simulink model "mechanics_with_estimation"  (R2014a)
settings: Solver=ode2  StartTime=0.0  StopTime=10  FixedStep=0.001  RelTol=1e-3
InitFcn:
  | estimation_initfcn
values from neighbouring files (symbols this model uses):
  c = [x y z]'    [estimation_initfcn.m]
  I_xx = 1/12*m*(y^2+z^2)    (= 0.00181666666667)    [estimation_initfcn.m]
  I_yy = 1/12*m*(x^2+z^2)    (= 0.0418166666667)    [estimation_initfcn.m]
  I_zz = 1/12*m*(y^2+x^2)    (= 0.0433333333333)    [estimation_initfcn.m]
  m = 2    [estimation_initfcn.m]
  x = 0.5    [estimation_initfcn.m]
  y = 0.1    [estimation_initfcn.m]
  z = 0.03    [estimation_initfcn.m]
undefined symbols (not defined in the file or in its folder): X, Y, Z
libraries: nesl_utility x16, sm_lib x11
settings Model: Creator=wirnshofer  LastModifiedBy=benediktibk

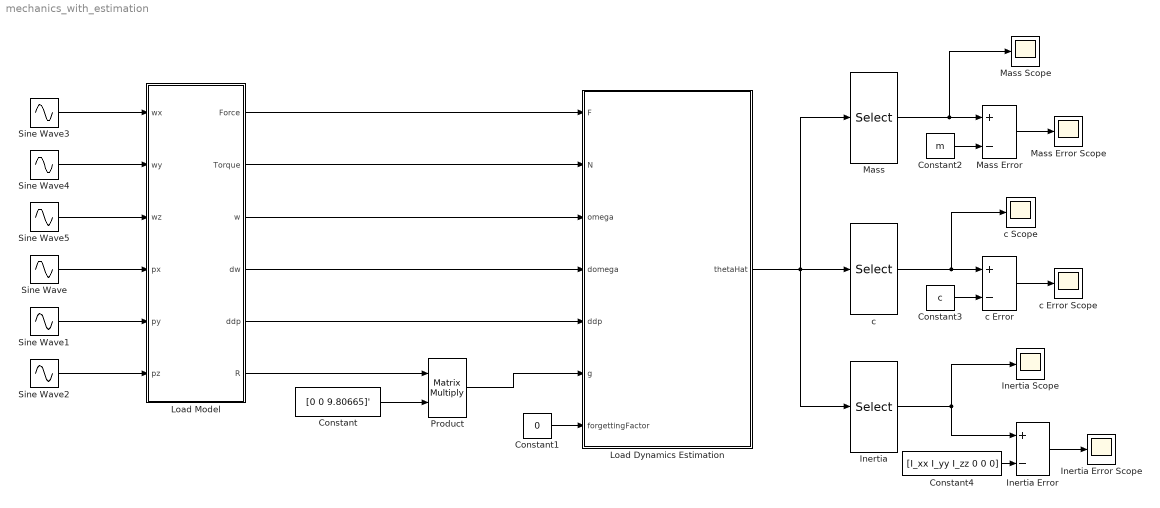
== system mechanics_with_estimation ==
  Constant : Constant  Value=[0 0 9.80665]'
  Constant1 : Constant  Value=0
  Constant2 : Constant  Value=m
  Constant3 : Constant  Value=c
  Constant4 : Constant  Value=[I_xx I_yy I_zz 0 0 0]
  Inertia : Selector  InputPortWidth=10  Indices=[5:10]
  Inertia Error : Sum  Inputs=+-
  Inertia Error Scope : Scope
      settings: ShowLegends=on  TimeRange=10  YMin=-0.9141621971570832  YMax=1.017206776816391  SaveName=ScopeData5
  Inertia Scope : Scope
      settings: ShowLegends=on  TimeRange=10  YMin=-1.003242729679008  YMax=1.975338173027628  SaveName=ScopeData2
  Load Dynamics Estimation : MATLAB Function  TreatAsAtomicUnit=on
  Load Model : Subsystem
  Mass : Selector  InputPortWidth=10
  Mass Error : Sum  Inputs=+-
  Mass Error Scope : Scope
      settings: ShowLegends=on  TimeRange=10  YMin=-0.2  YMax=0.15  SaveName=ScopeData3
  Mass Scope : Scope
      settings: ShowLegends=on  TimeRange=10  YMin=1.85  YMax=2.2
  Product : Product  Multiplication=Matrix(*)
  Sine Wave : Sin  Amplitude=0.2  Frequency=5  SampleTime=0
  Sine Wave1 : Sin  Amplitude=0.3  Frequency=4  SampleTime=0
  Sine Wave2 : Sin  Amplitude=0.2  Frequency=10  SampleTime=0
  Sine Wave3 : Sin  Amplitude=pi/4*1  Frequency=3  SampleTime=0
  Sine Wave4 : Sin  Amplitude=0.6  Frequency=8  SampleTime=0
  Sine Wave5 : Sin  Frequency=7  SampleTime=0
  c : Selector  InputPortWidth=10  Indices=[2:4]
  c Error : Sum  Inputs=+-
  c Error Scope : Scope
      settings: ShowLegends=on  TimeRange=10  YMin=-1.893593468040734  YMax=2.453897654456469  SaveName=ScopeData4
  c Scope : Scope
      settings: ShowLegends=on  TimeRange=10  YMin=-4.148671096345517  YMax=2.039036544850497
  wires:
  Constant/1 -> Product/2
  Product/1 -> Load Dynamics Estimation/6(g)
  Constant1/1 -> Load Dynamics Estimation/7(forgettingFactor)
  Sine Wave3/1 -> Load Model/1(wx)
  Sine Wave4/1 -> Load Model/2(wy)
  Sine Wave5/1 -> Load Model/3(wz)
  Sine Wave/1 -> Load Model/4(px)
  Sine Wave1/1 -> Load Model/5(py)
  Sine Wave2/1 -> Load Model/6(pz)
  Load Model/1(Force) -> Load Dynamics Estimation/1(F)
  Load Model/2(Torque) -> Load Dynamics Estimation/2(N)
  Load Model/3(w) -> Load Dynamics Estimation/3(omega)
  Load Model/4(dw) -> Load Dynamics Estimation/4(domega)
  Load Model/5(ddp) -> Load Dynamics Estimation/5(ddp)
  Load Model/6(R) -> Product/1
  Mass/1 -> Mass Error/1, Mass Scope/1
  Load Dynamics Estimation/1(thetaHat) -> Inertia/1, Mass/1, c/1
  c/1 -> c Error/1, c Scope/1
  Inertia/1 -> Inertia Error/1, Inertia Scope/1
  Constant2/1 -> Mass Error/2
  Mass Error/1 -> Mass Error Scope/1
  Constant3/1 -> c Error/2
  c Error/1 -> c Error Scope/1
  Constant4/1 -> Inertia Error/2
  Inertia Error/1 -> Inertia Error Scope/1

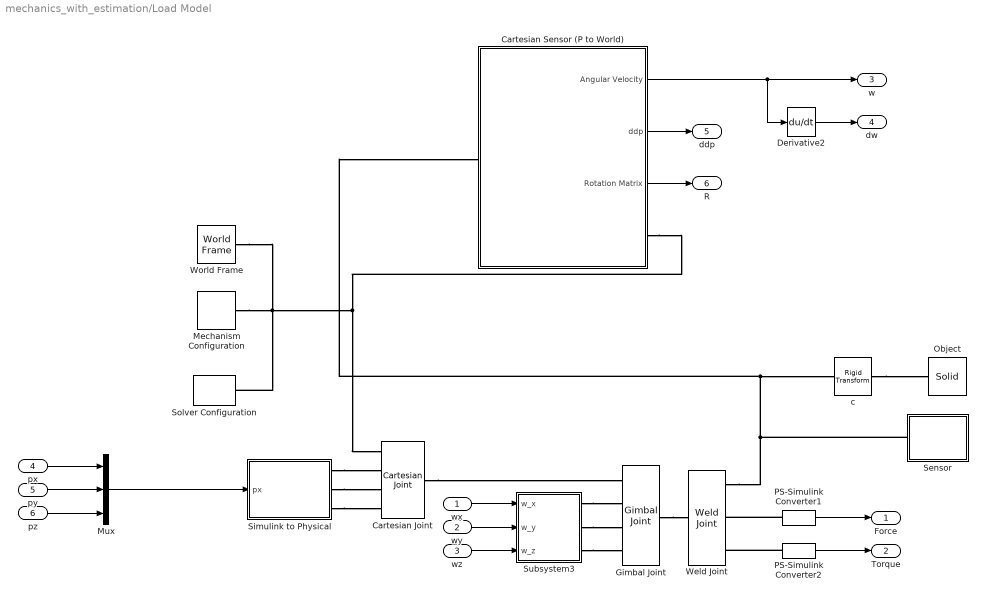
== system mechanics_with_estimation/Load Model ==
  wx : Inport
  wy : Inport  Port=2
  wz : Inport  Port=3
  px : Inport  Port=4
  py : Inport  Port=5
  pz : Inport  Port=6
  Cartesian Joint : sm_lib/Joints/Cartesian Joint  SenseConstraintForce=off  SenseConstraintForceX=off  SenseConstraintForceY=off  SenseConstraintForceZ=off  SenseConstraintTorque=off  SenseConstraintTorqueX=off  SenseConstraintTorqueY=off  SenseConstraintTorqueZ=off  SenseTotalForce=off  SenseTotalForceX=off  SenseTotalForceY=off  SenseTotalForceZ=off  SenseTotalTorque=off  SenseTotalTorqueX=off  SenseTotalTorqueY=off  SenseTotalTorqueZ=off  CompositeWrenchDir=FollowerOnBase  CompositeWrenchFrame=BaseFrame  PxEquilibriumPosition=0  PxEquilibriumPositionUnits=m  PxSpringStiffness=0  PxSpringStiffnessUnits=N/m  PxDampingCoefficient=0  PxDampingCoefficientUnits=N/(m/s)  PxTorqueActuationMode=ComputedTorque  PxMotionActuationMode=InputMotion  PxSensePosition=off  PxSenseVelocity=off  PxSenseAcceleration=off  PxSenseTorqueForce=off  PxPositionTargetValue=0  PxPositionTargetValueUnits=m  PxPositionTargetSpecify=off  PxPositionTargetPriority=High  PxVelocityTargetValue=0  PxVelocityTargetValueUnits=m/s  PxVelocityTargetSpecify=off  PxVelocityTargetPriority=High  PyEquilibriumPosition=0  PyEquilibriumPositionUnits=m  PySpringStiffness=0  PySpringStiffnessUnits=N/m  PyDampingCoefficient=0  PyDampingCoefficientUnits=N/(m/s)  PyTorqueActuationMode=ComputedTorque  PyMotionActuationMode=InputMotion  PySensePosition=off  PySenseVelocity=off  PySenseAcceleration=off  PySenseTorqueForce=off  PyPositionTargetValue=0  PyPositionTargetValueUnits=m  PyPositionTargetSpecify=off  PyPositionTargetPriority=High  PyVelocityTargetValue=0  PyVelocityTargetValueUnits=m/s  PyVelocityTargetSpecify=off  PyVelocityTargetPriority=High  PzEquilibriumPosition=0  PzEquilibriumPositionUnits=m  PzSpringStiffness=0  PzSpringStiffnessUnits=N/m  PzDampingCoefficient=0  PzDampingCoefficientUnits=N/(m/s)  PzTorqueActuationMode=ComputedTorque  PzMotionActuationMode=InputMotion  PzSensePosition=off  PzSenseVelocity=off  PzSenseAcceleration=off  PzSenseTorqueForce=off  PzPositionTargetValue=0  PzPositionTargetValueUnits=m  PzPositionTargetSpecify=off  PzPositionTargetPriority=High  PzVelocityTargetValue=0  PzVelocityTargetValueUnits=m/s  PzVelocityTargetSpecify=off  PzVelocityTargetPriority=High  BlockFunction=simmechanics.library.joints.cartesian_joint
  Cartesian Sensor (P to World) : Subsystem
  Derivative2 : Derivative
  Gimbal Joint : sm_lib/Joints/Gimbal Joint  SenseConstraintForce=off  SenseConstraintForceX=off  SenseConstraintForceY=off  SenseConstraintForceZ=off  SenseConstraintTorque=off  SenseConstraintTorqueX=off  SenseConstraintTorqueY=off  SenseConstraintTorqueZ=off  SenseTotalForce=off  SenseTotalForceX=off  SenseTotalForceY=off  SenseTotalForceZ=off  SenseTotalTorque=off  SenseTotalTorqueX=off  SenseTotalTorqueY=off  SenseTotalTorqueZ=off  CompositeWrenchDir=FollowerOnBase  CompositeWrenchFrame=BaseFrame  RxEquilibriumPosition=0  RxEquilibriumPositionUnits=deg  RxSpringStiffness=0  RxSpringStiffnessUnits=N*m/deg  RxDampingCoefficient=0  RxDampingCoefficientUnits=N*m/(deg/s)  RxTorqueActuationMode=ComputedTorque  RxMotionActuationMode=InputMotion  RxSensePosition=off  RxSenseVelocity=off  RxSenseAcceleration=off  RxSenseTorqueForce=off  RxPositionTargetValue=0  RxPositionTargetValueUnits=deg  RxPositionTargetSpecify=off  RxPositionTargetPriority=High  RxVelocityTargetValue=0  RxVelocityTargetValueUnits=deg/s  RxVelocityTargetSpecify=off  RxVelocityTargetPriority=High  RyEquilibriumPosition=0  RyEquilibriumPositionUnits=deg  RySpringStiffness=0  RySpringStiffnessUnits=N*m/deg  RyDampingCoefficient=0  RyDampingCoefficientUnits=N*m/(deg/s)  RyTorqueActuationMode=ComputedTorque  RyMotionActuationMode=InputMotion  RySensePosition=off  RySenseVelocity=off  RySenseAcceleration=off  RySenseTorqueForce=off  RyPositionTargetValue=0  RyPositionTargetValueUnits=deg  RyPositionTargetSpecify=off  RyPositionTargetPriority=High  RyVelocityTargetValue=0  RyVelocityTargetValueUnits=deg/s  RyVelocityTargetSpecify=off  RyVelocityTargetPriority=High  RzEquilibriumPosition=0  RzEquilibriumPositionUnits=deg  RzSpringStiffness=0  RzSpringStiffnessUnits=N*m/deg  RzDampingCoefficient=0  RzDampingCoefficientUnits=N*m/(deg/s)  RzTorqueActuationMode=ComputedTorque  RzMotionActuationMode=InputMotion  RzSensePosition=off  RzSenseVelocity=off  RzSenseAcceleration=off  RzSenseTorqueForce=off  RzPositionTargetValue=0  RzPositionTargetValueUnits=deg  RzPositionTargetSpecify=off  RzPositionTargetPriority=High  RzVelocityTargetValue=0  RzVelocityTargetValueUnits=deg/s  RzVelocityTargetSpecify=off  RzVelocityTargetPriority=High  BlockFunction=simmechanics.library.joints.gimbal_joint
  Mechanism Configuration : sm_lib/Utilities/Mechanism Configuration  UniformGravity=Constant  GravityVector=[0 0 -9.80665]  GravityUnits=m/s^2  LinearizationDelta=0.001  BlockFunction=simmechanics.library.utilities.mechanism_configuration
  Mux : Mux  Inputs=3
  Object : sm_lib/Body Elements/Solid  InertiaType=Custom  Mass=m  MassUnits=kg  CenterOfMass=[0 0 0]  CenterOfMassUnits=m  MomentsOfInertia=[I_xx I_yy I_zz]  MomentsOfInertiaUnits=kg*m^2  ProductsOfInertia=[0 0 0]  ProductsOfInertiaUnits=kg*m^2  DensityBased=on  Density=1000  DensityUnits=kg/(m^3)  GraphicType=FromGeometry  MarkerShape=Sphere  MarkerSize=10  MarkerSizeUnits=m  GraphicVisPropType=SimpleVisualProperties  GraphicDiffuseColor=[0.5 0.5 0.5]  GraphicSpecularColor=[0.5 0.5 0.5 1.0]  GraphicAmbientColor=[0.15 0.15 0.15 1.0]  GraphicEmissiveColor=[0.0 0.0 0.0 1.0]  GraphicShininess=75  GraphicOpacity=1.0  GeometryShape=Brick  RectangleSize=[1 1]  RectangleSizeUnits=m  BrickDimensions=[x y z]  BrickDimensionUnits=m  CylinderRadius=1  CylinderRadiusUnits=m  CylinderLength=1  CylinderLengthUnits=m  SphereRadius=1  SphereRadiusUnits=m  EllipsoidRadii=[1 1 1]  EllipsoidRadiiUnits=m  ExtrusionCrossSection=[1 1; -1 1; -1 -1; 1 -1]  ExtrusionCrossSectionUnits=m  ExtrusionLength=1  ExtrusionLengthUnits=m  PolygonNumSides=3  PolygonOuterRadius=1  PolygonOuterRadiusUnits=m  ExtGeomFileType=STL  ExtGeomFileUnits=m  RevolutionCrossSection=[1 1; 1 -1; 2 -1; 2 1]  RevolutionCrossSectionUnits=m  RevolutionExtent=Full  RevolutionAngle=180  RevolutionAngleUnits=deg  BlockFunction=simmechanics.library.body_elements.solid
  PS-Simulink Converter1 : nesl_utility/PS-Simulink Converter  PhysicalDomain=network_engine_domain  SubClassName=ps_output  LeftPortType=input  RightPortType=output  PseudoPeriodic=off  Frequencies=[]  Unit=1  AffineConversion=off
  PS-Simulink Converter2 : nesl_utility/PS-Simulink Converter  PhysicalDomain=network_engine_domain  SubClassName=ps_output  LeftPortType=input  RightPortType=output  PseudoPeriodic=off  Frequencies=[]  Unit=1  AffineConversion=off
  Sensor : Subsystem
  Simulink to Physical : Subsystem
  Solver Configuration : nesl_utility/Solver Configuration  PhysicalDomain=network_engine_domain  SubClassName=solver  LeftPortType=input  RightPortType=generic  Accelerate=off  Tones=[]  Harmonics=[]  SimulateNoise=off  Profile=off  UseLocalSampling=off  EnableSwitchedLinearOptims=on  FrequencyDomain=off  UseCCode=off  RelTol=0.001  AbsTol=1e-06  MinStep=1e-09  ToWorkspace=off  DoDC=off  ResidualTolerance=1e-09  UseLocalSolver=off  LocalSolverChoice=NE_BACKWARD_EULER_ADVANCER  LocalSolverSampleTime=0.001  DoFixedCost=off  MaxNonlinIter=3  MaxModeIter=2  LinearAlgebra=Sparse  DelaysMemoryBudget=1024  AutomaticFiltering=on  FilteringTimeConstant=0.001
  Subsystem3 : Subsystem
  Weld Joint : sm_lib/Joints/Weld Joint  SenseConstraintForce=off  SenseConstraintForceX=off  SenseConstraintForceY=off  SenseConstraintForceZ=off  SenseConstraintTorque=off  SenseConstraintTorqueX=off  SenseConstraintTorqueY=off  SenseConstraintTorqueZ=off  SenseTotalForce=on  SenseTotalForceX=off  SenseTotalForceY=off  SenseTotalForceZ=off  SenseTotalTorque=on  SenseTotalTorqueX=off  SenseTotalTorqueY=off  SenseTotalTorqueZ=off  CompositeWrenchDir=FollowerOnBase  CompositeWrenchFrame=BaseFrame  BlockFunction=simmechanics.library.joints.weld_joint
  World Frame : sm_lib/Frames and Transforms/World Frame  BlockFunction=simmechanics.library.frames_transforms.world_frame
  c : sm_lib/Frames and Transforms/Rigid Transform  TranslationMethod=Cartesian  TranslationLengthUnit=m  TranslationStandardAxis=+Z  TranslationStandardOffset=0  TranslationCartesianOffset=c  TranslationROffset=0  TranslationROffsetUnits=m  TranslationZOffset=0  TranslationZOffsetUnits=m  TranslationThetaOffset=0  TranslationThetaOffsetUnits=deg  RotationMethod=None  RotationAngleUnits=deg  RotationStandardAxis=+Z  RotationAngle=0  RotationArbitraryAxis=[0 0 1]  FollAlignAxisA=+X  BaseAlignAxisA=+Y  FollAlignAxisB=+Y  BaseAlignAxisB=+Z  BlockFunction=simmechanics.library.frames_transforms.rigid_transform
  Force : Outport
  Torque : Outport  Port=2
  w : Outport  Port=3
  dw : Outport  Port=4
  ddp : Outport  Port=5
  R : Outport  Port=6
  wires:
  px/1 -> Mux/1
  py/1 -> Mux/2
  pz/1 -> Mux/3
  wx/1 -> Subsystem3/1(w_x)
  wy/1 -> Subsystem3/2(w_y)
  wz/1 -> Subsystem3/3(w_z)
  Mux/1 -> Simulink to Physical/1(px)
  Derivative2/1 -> dw/1
  PS-Simulink Converter1/1 -> Force/1
  PS-Simulink Converter2/1 -> Torque/1
  Cartesian Sensor (P to World)/2(ddp) -> ddp/1
  Cartesian Sensor (P to World)/1(Angular Velocity) -> Derivative2/1, w/1
  Cartesian Sensor (P to World)/3(Rotation Matrix) -> R/1
  connections:
  Subsystem3/RConn1 -- Gimbal Joint/LConn2
  Subsystem3/RConn2 -- Gimbal Joint/LConn3
  Subsystem3/RConn3 -- Gimbal Joint/LConn4
  Cartesian Joint/RConn1 -- Gimbal Joint/LConn1
  Gimbal Joint/RConn1 -- Weld Joint/LConn1
  PS-Simulink Converter1/LConn1 -- Weld Joint/RConn2
  PS-Simulink Converter2/LConn1 -- Weld Joint/RConn3
  c/RConn1 -- Object/RConn1
  Solver Configuration/RConn1 -- World Frame/RConn1 -- Cartesian Sensor (P to World)/RConn1 -- Cartesian Joint/LConn1 -- Mechanism Configuration/RConn1
  Sensor/RConn1 -- Weld Joint/RConn1 -- Cartesian Sensor (P to World)/LConn1 -- c/LConn1
  Simulink to Physical/RConn2 -- Cartesian Joint/LConn3
  Simulink to Physical/RConn1 -- Cartesian Joint/LConn2
  Simulink to Physical/RConn3 -- Cartesian Joint/LConn4

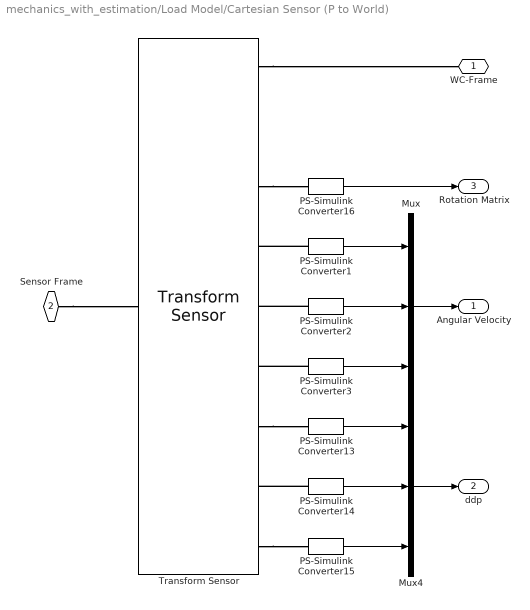
== system mechanics_with_estimation/Load Model/Cartesian Sensor (P to World) ==
  Mux : Mux  Inputs=3
  Mux4 : Mux  Inputs=3
  PS-Simulink Converter{1..3,13..16} (7 alike) : nesl_utility/PS-Simulink Converter  PhysicalDomain=network_engine_domain  SubClassName=ps_output  LeftPortType=input  RightPortType=output  PseudoPeriodic=off  Frequencies=[]  Unit=1  AffineConversion=off
  Transform Sensor : sm_lib/Frames and Transforms/Transform Sensor  MeasurementFrame=Base  SenseAngle=on  SenseAxis=off  SenseAngle1=off  SenseAngle2=off  SenseAngle3=off  SenseQ=off  SenseR=on  SenseOmegaX=on  SenseOmegaY=on  SenseOmegaZ=on  SenseOmega1=off  SenseOmega2=off  SenseOmega3=off  SenseQDot=off  SenseRDot=off  SenseAlphaX=off  SenseAlphaY=off  SenseAlphaZ=off  SenseAlpha1=off  SenseAlpha2=off  SenseAlpha3=off  SenseQDDot=off  SenseRDDot=off  SenseX=off  SenseY=off  SenseZ=off  SenseRad=off  SenseAzim=off  SenseDist=off  SenseInc=off  SenseXDot=off  SenseYDot=off  SenseZDot=off  SenseRadDot=off  SenseAzimDot=off  SenseDistDot=off  SenseIncDot=off  SenseXDDot=on  SenseYDDot=on  SenseZDDot=on  SenseRadDDot=off  SenseAzimDDot=off  SenseDistDDot=off  SenseIncDDot=off  BlockFunction=simmechanics.library.frames_transforms.transform_sensor
  WC-Frame : PMIOPort  Port=1  Side=Right
  Sensor Frame : PMIOPort  Port=2  Side=Left
  Angular Velocity : Outport
  ddp : Outport  Port=2
  Rotation Matrix : Outport  Port=3
  wires:
  PS-Simulink Converter2/1 -> Mux/2
  PS-Simulink Converter1/1 -> Mux/1
  Mux/1 -> Angular Velocity/1
  PS-Simulink Converter3/1 -> Mux/3
  PS-Simulink Converter14/1 -> Mux4/2
  Mux4/1 -> ddp/1
  PS-Simulink Converter15/1 -> Mux4/3
  PS-Simulink Converter13/1 -> Mux4/1
  PS-Simulink Converter16/1 -> Rotation Matrix/1
  connections:
  Transform Sensor/RConn1 -- WC-Frame/RConn1
  Sensor Frame/RConn1 -- Transform Sensor/LConn1
  PS-Simulink Converter2/LConn1 -- Transform Sensor/RConn5
  PS-Simulink Converter1/LConn1 -- Transform Sensor/RConn4
  PS-Simulink Converter3/LConn1 -- Transform Sensor/RConn6
  PS-Simulink Converter14/LConn1 -- Transform Sensor/RConn8
  Transform Sensor/RConn7 -- PS-Simulink Converter13/LConn1
  Transform Sensor/RConn9 -- PS-Simulink Converter15/LConn1
  Transform Sensor/RConn3 -- PS-Simulink Converter16/LConn1

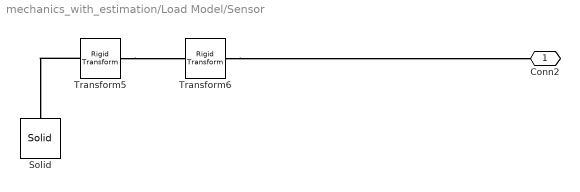
== system mechanics_with_estimation/Load Model/Sensor ==
  Solid : sm_lib/Body Elements/Solid  InertiaType=CalculateFromGeometry  Mass=0.000000000001  MassUnits=kg  CenterOfMass=[0 0 0]  CenterOfMassUnits=m  MomentsOfInertia=[1 1 1]  MomentsOfInertiaUnits=kg*m^2  ProductsOfInertia=[0 0 0]  ProductsOfInertiaUnits=kg*m^2  DensityBased=off  Density=1000  DensityUnits=kg/(m^3)  GraphicType=FromGeometry  MarkerShape=Sphere  MarkerSize=10  MarkerSizeUnits=m  GraphicVisPropType=SimpleVisualProperties  GraphicDiffuseColor=[0.0 0.0 1.0]  GraphicSpecularColor=[0.5 0.5 0.5 1.0]  GraphicAmbientColor=[0.15 0.15 0.15 1.0]  GraphicEmissiveColor=[0.0 0.0 0.0 1.0]  GraphicShininess=75  GraphicOpacity=1.0  GeometryShape=Cylinder  RectangleSize=[1 1]  RectangleSizeUnits=m  BrickDimensions=[1 1 1]  BrickDimensionUnits=m  CylinderRadius=0.025  CylinderRadiusUnits=m  CylinderLength=0.03  CylinderLengthUnits=m  SphereRadius=1  SphereRadiusUnits=m  EllipsoidRadii=[1 1 1]  EllipsoidRadiiUnits=m  ExtrusionCrossSection=[1 1; -1 1; -1 -1; 1 -1]  ExtrusionCrossSectionUnits=m  ExtrusionLength=1  ExtrusionLengthUnits=m  PolygonNumSides=3  PolygonOuterRadius=1  PolygonOuterRadiusUnits=m  ExtGeomFileType=STL  ExtGeomFileUnits=m  RevolutionCrossSection=[1 1; 1 -1; 2 -1; 2 1]  RevolutionCrossSectionUnits=m  RevolutionExtent=Full  RevolutionAngle=180  RevolutionAngleUnits=deg  BlockFunction=simmechanics.library.body_elements.solid
  Transform5 : sm_lib/Frames and Transforms/Rigid Transform  TranslationMethod=None  TranslationLengthUnit=mm  TranslationStandardAxis=+Z  TranslationStandardOffset=0  TranslationCartesianOffset=[0 0 0]  TranslationROffset=0  TranslationROffsetUnits=m  TranslationZOffset=0  TranslationZOffsetUnits=m  TranslationThetaOffset=0  TranslationThetaOffsetUnits=deg  RotationMethod=StandardAxis  RotationAngleUnits=deg  RotationStandardAxis=+Y  RotationAngle=90  RotationArbitraryAxis=[0 0 1]  FollAlignAxisA=+X  BaseAlignAxisA=+Y  FollAlignAxisB=+Y  BaseAlignAxisB=+Z  BlockFunction=simmechanics.library.frames_transforms.rigid_transform
  Transform6 : sm_lib/Frames and Transforms/Rigid Transform  TranslationMethod=Cartesian  TranslationLengthUnit=m  TranslationStandardAxis=+Z  TranslationStandardOffset=0  TranslationCartesianOffset=[0.015 0 0]  TranslationROffset=0  TranslationROffsetUnits=m  TranslationZOffset=0  TranslationZOffsetUnits=m  TranslationThetaOffset=0  TranslationThetaOffsetUnits=deg  RotationMethod=None  RotationAngleUnits=deg  RotationStandardAxis=+Z  RotationAngle=0  RotationArbitraryAxis=[0 0 1]  FollAlignAxisA=+X  BaseAlignAxisA=+Y  FollAlignAxisB=+Y  BaseAlignAxisB=+Z  BlockFunction=simmechanics.library.frames_transforms.rigid_transform
  Conn2 : PMIOPort  Port=1  Side=Right
  connections:
  Transform5/LConn1 -- Solid/RConn1
  Transform6/RConn1 -- Conn2/RConn1
  Transform5/RConn1 -- Transform6/LConn1

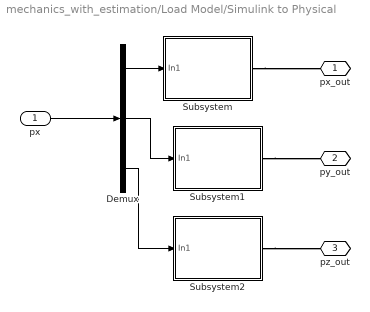
== system mechanics_with_estimation/Load Model/Simulink to Physical ==
  px : Inport
  Demux : Demux  Outputs=3
  Subsystem : Subsystem
  Subsystem1 : Subsystem
  Subsystem2 : Subsystem
  px_out : PMIOPort  Port=1  Side=Right
  py_out : PMIOPort  Port=2  Side=Right
  pz_out : PMIOPort  Port=3  Side=Right
  wires:
  px/1 -> Demux/1
  Demux/1 -> Subsystem/1(In1)
  Demux/2 -> Subsystem1/1(In1)
  Demux/3 -> Subsystem2/1(In1)
  connections:
  Subsystem2/RConn1 -- pz_out/RConn1
  Subsystem/RConn1 -- px_out/RConn1
  Subsystem1/RConn1 -- py_out/RConn1

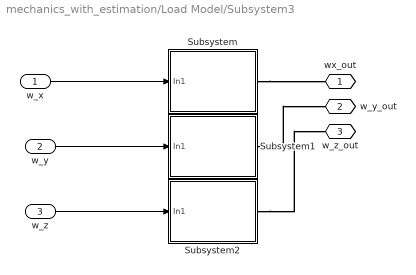
== system mechanics_with_estimation/Load Model/Subsystem3 ==
  w_x : Inport
  w_y : Inport  Port=2
  w_z : Inport  Port=3
  Subsystem : Subsystem
  Subsystem1 : Subsystem
  Subsystem2 : Subsystem
  wx_out : PMIOPort  Port=1  Side=Right
  w_y_out : PMIOPort  Port=2  Side=Right
  w_z_out : PMIOPort  Port=3  Side=Right
  wires:
  w_z/1 -> Subsystem2/1(In1)
  w_y/1 -> Subsystem1/1(In1)
  w_x/1 -> Subsystem/1(In1)
  connections:
  Subsystem1/RConn1 -- w_y_out/RConn1
  Subsystem/RConn1 -- wx_out/RConn1
  Subsystem2/RConn1 -- w_z_out/RConn1

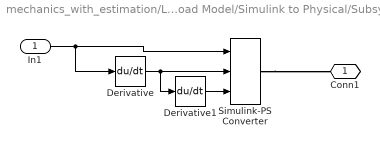
== system mechanics_with_estimation/Load Model/Simulink to Physical/Subsystem ==
  In1 : Inport
  Derivative : Derivative
  Derivative1 : Derivative
  Simulink-PS Converter : nesl_utility/Simulink-PS Converter  PhysicalDomain=network_engine_domain  SubClassName=ps_input  LeftPortType=input  RightPortType=output  PseudoPeriodic=off  Frequencies=[]  NoiseDistribution=none  NoiseParameters=[]  Unit=1  AffineConversion=off  InputFiltering=derivs  SimscapeFilterOrder=1  InputFilterTimeConstant=0.001  UdotUserProvided=2
  Conn1 : PMIOPort  Port=1  Side=Right
  wires:
  Derivative1/1 -> Simulink-PS Converter/3
  Derivative/1 -> Simulink-PS Converter/2, Derivative1/1
  In1/1 -> Derivative/1, Simulink-PS Converter/1
  connections:
  Simulink-PS Converter/RConn1 -- Conn1/RConn1

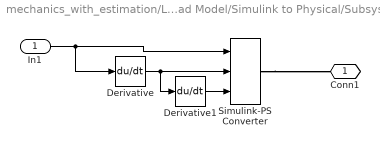
== system mechanics_with_estimation/Load Model/Simulink to Physical/Subsystem1 ==
  In1 : Inport
  Derivative : Derivative
  Derivative1 : Derivative
  Simulink-PS Converter : nesl_utility/Simulink-PS Converter  PhysicalDomain=network_engine_domain  SubClassName=ps_input  LeftPortType=input  RightPortType=output  PseudoPeriodic=off  Frequencies=[]  NoiseDistribution=none  NoiseParameters=[]  Unit=1  AffineConversion=off  InputFiltering=derivs  SimscapeFilterOrder=1  InputFilterTimeConstant=0.001  UdotUserProvided=2
  Conn1 : PMIOPort  Port=1  Side=Right
  wires:
  Derivative1/1 -> Simulink-PS Converter/3
  Derivative/1 -> Simulink-PS Converter/2, Derivative1/1
  In1/1 -> Derivative/1, Simulink-PS Converter/1
  connections:
  Simulink-PS Converter/RConn1 -- Conn1/RConn1

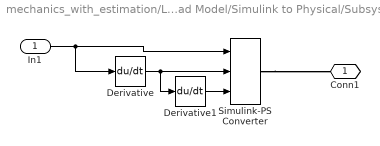
== system mechanics_with_estimation/Load Model/Simulink to Physical/Subsystem2 ==
  In1 : Inport
  Derivative : Derivative
  Derivative1 : Derivative
  Simulink-PS Converter : nesl_utility/Simulink-PS Converter  PhysicalDomain=network_engine_domain  SubClassName=ps_input  LeftPortType=input  RightPortType=output  PseudoPeriodic=off  Frequencies=[]  NoiseDistribution=none  NoiseParameters=[]  Unit=1  AffineConversion=off  InputFiltering=derivs  SimscapeFilterOrder=1  InputFilterTimeConstant=0.001  UdotUserProvided=2
  Conn1 : PMIOPort  Port=1  Side=Right
  wires:
  Derivative1/1 -> Simulink-PS Converter/3
  Derivative/1 -> Simulink-PS Converter/2, Derivative1/1
  In1/1 -> Derivative/1, Simulink-PS Converter/1
  connections:
  Simulink-PS Converter/RConn1 -- Conn1/RConn1

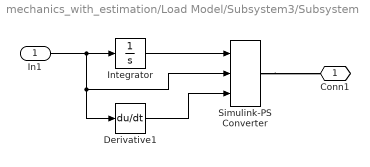
== system mechanics_with_estimation/Load Model/Subsystem3/Subsystem ==
  In1 : Inport
  Derivative1 : Derivative
  Integrator : Integrator
  Simulink-PS Converter : nesl_utility/Simulink-PS Converter  PhysicalDomain=network_engine_domain  SubClassName=ps_input  LeftPortType=input  RightPortType=output  PseudoPeriodic=off  Frequencies=[]  NoiseDistribution=none  NoiseParameters=[]  Unit=1  AffineConversion=off  InputFiltering=derivs  SimscapeFilterOrder=1  InputFilterTimeConstant=0.001  UdotUserProvided=2
  Conn1 : PMIOPort  Port=1  Side=Right
  wires:
  Derivative1/1 -> Simulink-PS Converter/3
  In1/1 -> Simulink-PS Converter/2, Derivative1/1, Integrator/1
  Integrator/1 -> Simulink-PS Converter/1
  connections:
  Simulink-PS Converter/RConn1 -- Conn1/RConn1

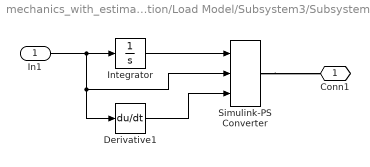
== system mechanics_with_estimation/Load Model/Subsystem3/Subsystem1 ==
  In1 : Inport
  Derivative1 : Derivative
  Integrator : Integrator
  Simulink-PS Converter : nesl_utility/Simulink-PS Converter  PhysicalDomain=network_engine_domain  SubClassName=ps_input  LeftPortType=input  RightPortType=output  PseudoPeriodic=off  Frequencies=[]  NoiseDistribution=none  NoiseParameters=[]  Unit=1  AffineConversion=off  InputFiltering=derivs  SimscapeFilterOrder=1  InputFilterTimeConstant=0.001  UdotUserProvided=2
  Conn1 : PMIOPort  Port=1  Side=Right
  wires:
  Derivative1/1 -> Simulink-PS Converter/3
  In1/1 -> Simulink-PS Converter/2, Derivative1/1, Integrator/1
  Integrator/1 -> Simulink-PS Converter/1
  connections:
  Simulink-PS Converter/RConn1 -- Conn1/RConn1

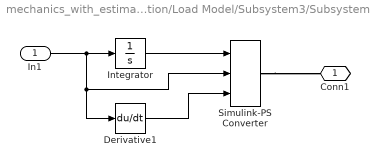
== system mechanics_with_estimation/Load Model/Subsystem3/Subsystem2 ==
  In1 : Inport
  Derivative1 : Derivative
  Integrator : Integrator
  Simulink-PS Converter : nesl_utility/Simulink-PS Converter  PhysicalDomain=network_engine_domain  SubClassName=ps_input  LeftPortType=input  RightPortType=output  PseudoPeriodic=off  Frequencies=[]  NoiseDistribution=none  NoiseParameters=[]  Unit=1  AffineConversion=off  InputFiltering=derivs  SimscapeFilterOrder=1  InputFilterTimeConstant=0.001  UdotUserProvided=2
  Conn1 : PMIOPort  Port=1  Side=Right
  wires:
  Derivative1/1 -> Simulink-PS Converter/3
  In1/1 -> Simulink-PS Converter/2, Derivative1/1, Integrator/1
  Integrator/1 -> Simulink-PS Converter/1
  connections:
  Simulink-PS Converter/RConn1 -- Conn1/RConn1

== matlab function mechanics_with_estimation/Load Dynamics Estimation ==
  data: F input; thetaHat output; N input; omega input; domega input; ddp input; g input; forgettingFactor input
function thetaHat = fcn(F,N,omega,domega,ddp,g,forgettingFactor)
persistent thetaHatPrevious PPrevious initializationNecessary;

if isempty(initializationNecessary)
    initializationNecessary = 1;
end

% calculate linear relation Phi between the estimates and the input
omegaCross = crossMatrix(omega);
domegaCross = crossMatrix(domega);
omegaDot = dotMatrix(omega);
domegaDot = dotMatrix(domega);
h = [F;N];
Phi = [ddp-g , domegaCross+omegaCross*omegaCross, zeros(3,6) ; zeros(3,1) , crossMatrix(g-ddp) , domegaDot+omegaCross*omegaDot];

% intialize persisent variables
if initializationNecessary == 1 || isempty(PPrevious)
    PPrevious = inv(Phi'*Phi);
    thetaHatPrevious = PPrevious*Phi'*h;
    thetaHat = thetaHatPrevious;
    initializationNecessary = 0;
    return;
end    

% check for invalid values in the current state
if any(any(isnan(PPrevious)))
    initializationNecessary = 1;
    thetaHat = thetaHatPrevious;
    return;  
end    

KInternal = eye(6)+Phi*PPrevious*Phi';
KInternalInv = inv(KInternal);

% check for invalid values in the current estimation step
if calculateConditionDistance(KInternal, KInternalInv) > 1e20
    initializationNecessary = 1;
    thetaHat = thetaHatPrevious;
    return;  
end

% calculate improved estimation
K = PPrevious*Phi'*KInternalInv;
PNew = (eye(10)-K*Phi)*PPrevious;
P = (1 - forgettingFactor)*PNew + forgettingFactor*PPrevious;
thetaHatNew = thetaHatPrevious+K*(h-Phi*thetaHatPrevious);
thetaHat = (1 - forgettingFactor)*thetaHatNew + forgettingFactor*thetaHatPrevious;
PPrevious = P;
thetaHatPrevious = thetaHat;
